simulink model "s_spg_pp"  (Simulink 8.1)
settings: Solver=ode4  SolverMode=SingleTasking  StartTime=0.0  StopTime=15  FixedStep=0.002  RelTol=1e-3  AbsTol=1e-6
values from neighbouring files (symbols this model uses):
  Beq = 5.4    [setup_ip01_2_configuration.m]
  Eff_g = 1    [setup_ip01_2_configuration.m]
  Eff_m = 1    [setup_ip01_2_configuration.m]
  IMAX_UPM = 3    [setup_ip01_2_configuration.m]
  K = place( A, B, cl_poles )    [d_ip02_spg_pp.m]    (also in prelab2_k_values.m = place (Ai,Bi,[p1, p2, p3, p4, p5]); setup_lab_ip02_spg.m = [ 0 0 0 0 ])
  Kg = 3.71    [setup_ip01_2_configuration.m]
  Km = 0.804e-3 * K_RDPS2RPM    [setup_ip01_2_configuration.m]
  Kt = 1.088 * K_OZ2N * K_IN2M    [setup_ip01_2_configuration.m]
  Mc = Mc + Eff_g * Kg^2 * Jm / r_mp^2    [setup_lab_ip02_spg.m]
  r_mp = 0.5 / 2 * K_IN2M    [setup_ip01_2_configuration.m]
  Rm = 2.6    [setup_ip01_2_configuration.m]
  VMAX_UPM = 13    [setup_ip01_2_configuration.m]
  X0 = [ 0; X0(2); 0; 0 ]    [setup_lab_ip02_spg.m]
undefined symbols (not defined in the file or in its folder): Bp, g, Ip, lp, Lp, Mp
libraries: simulink_extras x1
settings Model: Creator=Willdog  LastModifiedBy=Willdog  ExtModeArmWhenConnect=off  ExtModeAutoUpdateStatusClock=off  BufferReuse=off
settings DataIOCC: LimitDataPoints=off
settings OptimizationCC: BooleanDataType=off  OptimizeBlockIOStorage=off  BufferReuse=off  ExpressionFolding=off  ExpressionDepthLimit=128  FoldNonRolledExpr=off  LocalBlockOutputs=off  InitFltsAndDblsToZero=on
settings DebuggingCC: SaveWithParameterizedLinksMsg=none  SignalResolutionControl=TryResolveAllWithWarning  SolverPrmCheckMsg=none  MultiTaskDSMMsg=warning  MultiTaskCondExecSysMsg=none  StrictBusMsg=None
settings RTWCC: SystemTargetFile=wincon.tlc  MakeCommand=make_wc  TemplateMakefile=nt_msvc.tmf  Description=WinCon Target  ProcessScript=wincon_make_rtw_hook  IncludeERTFirstTime=on
settings STFCustomTargetCC: TargetFcnLib=ansi_tfl_tmw.mat  CodeReplacementLibrary=ANSI_C  ModelReferenceCompliant=off  GeneratePreprocessorConditionals=Disable all  SystemTargetFile=wincon.tlc
settings GRTTargetCC: TargetFcnLib=ansi_tfl_tmw.mat  ModelReferenceCompliant=off  ParMdlRefBuildCompliant=off  CompOptLevelCompliant=off  ConcurrentExecutionCompliant=off  MatFileLogging=off  ExtMode=on
settings CustomProperty: Value=on

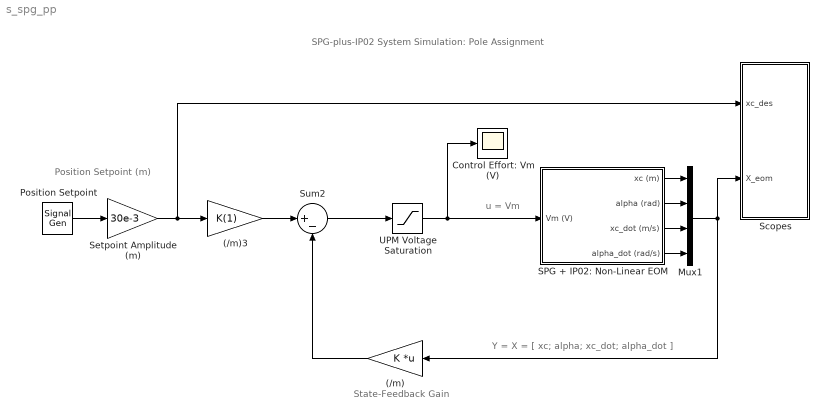
== system s_spg_pp ==
  note: u = Vm
  note: Y = X = [ xc; alpha; xc_dot; alpha_dot ]
  note: State-Feedback Gain
  note: Position Setpoint (m)
  note: SPG-plus-IP02 System Simulation:
      | Pole Assignment
  (/m) : Gain  Gain=K  Multiplication=Matrix(K*u)  SaturateOnIntegerOverflow=on  OutDataTypeStr=Inherit: Same as input  ParamDataTypeStr=Inherit: Same as input
  (/m)3 : Gain  Gain=K(1)  SaturateOnIntegerOverflow=on  OutDataTypeStr=Inherit: Same as input  ParamDataTypeStr=Inherit: Same as input
  Control Effort: Vm (V) : Scope
      settings: TickLabels=on  TimeRange=5  YMin=-35  YMax=35  SaveName=ScopeData2
  Mux1 : Mux
  Position Setpoint : SignalGenerator  WaveForm=square  Amplitude=0  Frequency=0.1
  SPG + IP02: Non-Linear EOM : Subsystem
  Scopes : Subsystem
  Setpoint Amplitude (m) : Gain  Gain=30e-3  SaturateOnIntegerOverflow=on  OutDataTypeStr=Inherit: Same as input  ParamDataTypeStr=Inherit: Same as input
  Sum2 : Sum  Inputs=|+-  SaturateOnIntegerOverflow=on  InputSameDT=on  OutDataTypeStr=Inherit: Same as first input
  UPM Voltage Saturation : Saturate  UpperLimit=VMAX_UPM  LowerLimit=- VMAX_UPM
  wires:
  UPM Voltage Saturation/1 -> Control Effort: Vm (V)/1, SPG + IP02: Non-Linear EOM/1(Vm (V))
  (/m)3/1 -> Sum2/1
  Setpoint Amplitude (m)/1 -> Scopes/1(xc_des), (/m)3/1
  Position Setpoint/1 -> Setpoint Amplitude (m)/1
  Mux1/1 -> Scopes/2(X_eom), (/m)/1
  (/m)/1 -> Sum2/2
  SPG + IP02: Non-Linear EOM/1(xc (m)) -> Mux1/1
  SPG + IP02: Non-Linear EOM/2(alpha (rad)) -> Mux1/2
  SPG + IP02: Non-Linear EOM/3(xc_dot (m/s)) -> Mux1/3
  SPG + IP02: Non-Linear EOM/4(alpha_dot (rad/s)) -> Mux1/4
  Sum2/1 -> UPM Voltage Saturation/1

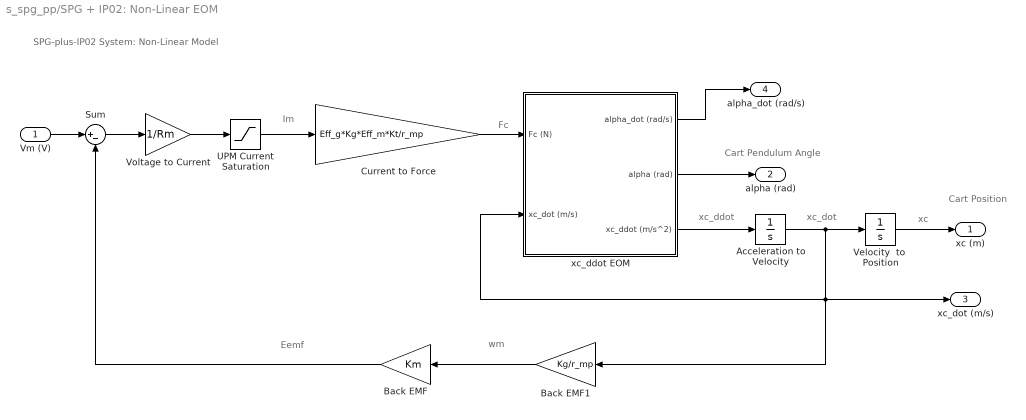
== system s_spg_pp/SPG + IP02: Non-Linear EOM ==
  note: SPG-plus-IP02 System:
      | Non-Linear Model
  note: Fc
  note: Im
  note: Eemf
  note: wm
  note: xc_dot
  note: xc_ddot
  note: xc
  note: Cart Position
  note: Cart Pendulum Angle
  Vm (V) : Inport
  Acceleration to Velocity : Integrator  InitialCondition=X0(3)
  Back EMF : Gain  Gain=Km  SaturateOnIntegerOverflow=on  OutDataTypeStr=Inherit: Same as input  ParamDataTypeStr=Inherit: Same as input
  Back EMF1 : Gain  Gain=Kg/r_mp  SaturateOnIntegerOverflow=on  OutDataTypeStr=Inherit: Same as input  ParamDataTypeStr=Inherit: Same as input
  Current to Force : Gain  Gain=Eff_g*Kg*Eff_m*Kt/r_mp  SaturateOnIntegerOverflow=on  OutDataTypeStr=Inherit: Same as input  ParamDataTypeStr=Inherit: Same as input
  Sum : Sum  Inputs=|+-  SaturateOnIntegerOverflow=on  InputSameDT=on  OutDataTypeStr=Inherit: Same as first input
  "UPM Current Saturation " : Saturate  UpperLimit=IMAX_UPM  LowerLimit=- IMAX_UPM
  Velocity  to  Position : Integrator  InitialCondition=X0(1)
  Voltage to Current : Gain  Gain=1/Rm  SaturateOnIntegerOverflow=on  OutDataTypeStr=Inherit: Same as input  ParamDataTypeStr=Inherit: Same as input
  xc_ddot EOM : Subsystem
  xc (m) : Outport
  alpha (rad) : Outport  Port=2
  xc_dot (m/s) : Outport  Port=3  InitialOutput=0
  alpha_dot (rad/s) : Outport  Port=4  InitialOutput=0
  wires:
  Sum/1 -> Voltage to Current/1
  Voltage to Current/1 -> "UPM Current Saturation "/1
  Acceleration to Velocity/1 -> xc_dot (m/s)/1, Back EMF1/1, xc_ddot EOM/2(xc_dot (m/s)), Velocity  to  Position/1
  Back EMF1/1 -> Back EMF/1
  Vm (V)/1 -> Sum/1
  Velocity  to  Position/1 -> xc (m)/1
  Back EMF/1 -> Sum/2
  "UPM Current Saturation "/1 -> Current to Force/1
  Current to Force/1 -> xc_ddot EOM/1(Fc (N))
  xc_ddot EOM/3(xc_ddot (m/s^2)) -> Acceleration to Velocity/1
  xc_ddot EOM/2(alpha (rad)) -> alpha (rad)/1
  xc_ddot EOM/1(alpha_dot (rad/s)) -> alpha_dot (rad/s)/1

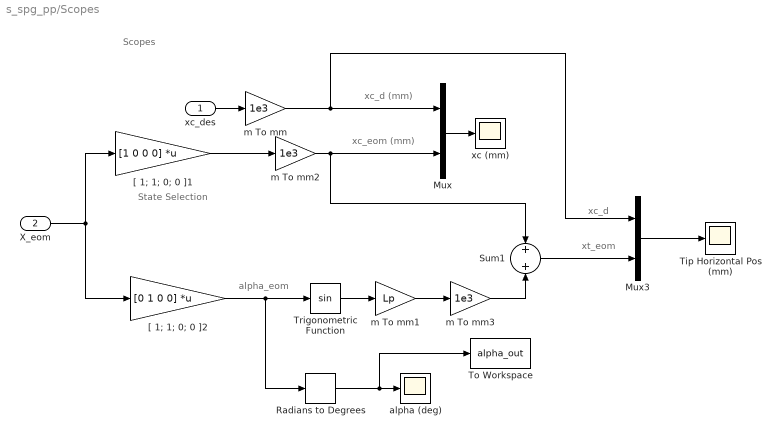
== system s_spg_pp/Scopes ==
  note: Scopes
  note: xc_d (mm)
  note: alpha_eom
  note: State Selection
  note: xc_eom (mm)
  note: xc_d
  note: xt_eom
  xc_des : Inport
  X_eom : Inport  Port=2
  Mux : Mux  Inputs=2
  Mux3 : Mux  Inputs=2
  Radians to Degrees : simulink_extras/Transformations/Radians to Degrees
  Sum1 : Sum  Inputs=+|+  SaturateOnIntegerOverflow=on  InputSameDT=on  OutDataTypeStr=Inherit: Same as first input
  Tip Horizontal Pos (mm) : Scope
      settings: SaveName=ScopeData5
  To Workspace : ToWorkspace  VariableName=alpha_out  SampleTime=-1  SaveFormat=Timeseries
  Trigonometric Function : Trigonometry
  "[ 1; 1; 0; 0 ]1" : Gain  Gain=[1 0 0 0]  Multiplication=Matrix(K*u)  SaturateOnIntegerOverflow=on  OutDataTypeStr=Inherit: Same as input  ParamDataTypeStr=Inherit: Same as input
  "[ 1; 1; 0; 0 ]2" : Gain  Gain=[0 1 0 0]  Multiplication=Matrix(K*u)  SaturateOnIntegerOverflow=on  OutDataTypeStr=Inherit: Same as input  ParamDataTypeStr=Inherit: Same as input
  alpha (deg) : Scope
      settings: TickLabels=on  TimeRange=1.000000  YMin=-250  YMax=250  SaveName=ScopeData3
  m To mm : Gain  Gain=1e3  SaturateOnIntegerOverflow=on  OutDataTypeStr=Inherit: Same as input  ParamDataTypeStr=Inherit: Same as input
  m To mm1 : Gain  Gain=Lp  SaturateOnIntegerOverflow=on  OutDataTypeStr=Inherit: Same as input  ParamDataTypeStr=Inherit: Same as input
  m To mm2 : Gain  Gain=1e3  SaturateOnIntegerOverflow=on  OutDataTypeStr=Inherit: Same as input  ParamDataTypeStr=Inherit: Same as input
  m To mm3 : Gain  Gain=1e3  SaturateOnIntegerOverflow=on  OutDataTypeStr=Inherit: Same as input  ParamDataTypeStr=Inherit: Same as input
  xc (mm) : Scope
      settings: TickLabels=on  TimeRange=5  YMin=-35  YMax=35
  wires:
  "[ 1; 1; 0; 0 ]2"/1 -> Radians to Degrees/1, Trigonometric Function/1
  X_eom/1 -> "[ 1; 1; 0; 0 ]2"/1, "[ 1; 1; 0; 0 ]1"/1
  xc_des/1 -> m To mm/1
  "[ 1; 1; 0; 0 ]1"/1 -> m To mm2/1
  Mux/1 -> xc (mm)/1
  m To mm1/1 -> m To mm3/1
  Trigonometric Function/1 -> m To mm1/1
  m To mm3/1 -> Sum1/2
  Radians to Degrees/1 -> To Workspace/1, alpha (deg)/1
  Mux3/1 -> Tip Horizontal Pos (mm)/1
  Sum1/1 -> Mux3/2
  m To mm/1 -> Mux/1, Mux3/1
  m To mm2/1 -> Mux/2, Sum1/1

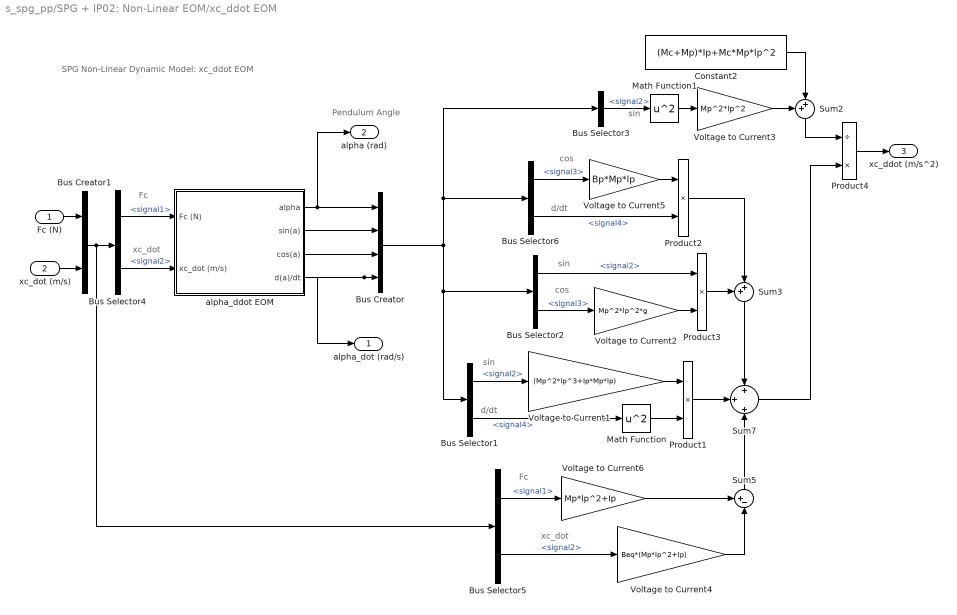
== system s_spg_pp/SPG + IP02: Non-Linear EOM/xc_ddot EOM ==
  note: d/dt
  note: sin
  note: sin
  note: cos
  note: sin
  note: Pendulum Angle
  note: cos
  note: d/dt
  note: Fc
  note: xc_dot
  note: Fc
  note: xc_dot
  note: SPG Non-Linear Dynamic Model:
      | xc_ddot EOM
  Fc (N) : Inport
  xc_dot (m/s) : Inport  Port=2
  Bus Creator : BusCreator
  Bus Creator1 : BusCreator  Inputs=2
  Bus Selector1 : BusSelector  OutputSignals=signal2,signal4
  Bus Selector2 : BusSelector  OutputSignals=signal2,signal3
  Bus Selector3 : BusSelector  OutputSignals=signal2
  Bus Selector4 : BusSelector  OutputSignals=signal1,signal2
  Bus Selector5 : BusSelector  OutputSignals=signal1,signal2
  Bus Selector6 : BusSelector  OutputSignals=signal3,signal4
  Constant2 : Constant  Value=(Mc+Mp)*Ip+Mc*Mp*lp^2
  Math Function : Math  Operator=square  SaturateOnIntegerOverflow=on
  Math Function1 : Math  Operator=square  SaturateOnIntegerOverflow=on
  Product1 : Product  SaturateOnIntegerOverflow=on  RndMeth=Zero  InputSameDT=on  OutDataTypeStr=Inherit: Same as first input
  Product2 : Product  SaturateOnIntegerOverflow=on  RndMeth=Zero  InputSameDT=on  OutDataTypeStr=Inherit: Same as first input
  Product3 : Product  SaturateOnIntegerOverflow=on  RndMeth=Zero  InputSameDT=on  OutDataTypeStr=Inherit: Same as first input
  Product4 : Product  Inputs=/*  SaturateOnIntegerOverflow=on  RndMeth=Zero  InputSameDT=on  OutDataTypeStr=Inherit: Same as first input
  Sum2 : Sum  Inputs=++|  SaturateOnIntegerOverflow=on  InputSameDT=on  OutDataTypeStr=Inherit: Same as first input
  Sum3 : Sum  Inputs=++|  SaturateOnIntegerOverflow=on  InputSameDT=on  OutDataTypeStr=Inherit: Same as first input
  Sum5 : Sum  Inputs=+-|  SaturateOnIntegerOverflow=on  InputSameDT=on  OutDataTypeStr=Inherit: Same as first input
  Sum7 : Sum  Inputs=+|+|+  SaturateOnIntegerOverflow=on  InputSameDT=on  OutDataTypeStr=Inherit: Same as first input
  Voltage to Current1 : Gain  Gain=(Mp^2*lp^3+Ip*Mp*lp)  SaturateOnIntegerOverflow=on  OutDataTypeStr=Inherit: Same as input  ParamDataTypeStr=Inherit: Same as input
  Voltage to Current2 : Gain  Gain=Mp^2*lp^2*g  SaturateOnIntegerOverflow=on  OutDataTypeStr=Inherit: Same as input  ParamDataTypeStr=Inherit: Same as input
  Voltage to Current3 : Gain  Gain=Mp^2*lp^2  SaturateOnIntegerOverflow=on  OutDataTypeStr=Inherit: Same as input  ParamDataTypeStr=Inherit: Same as input
  Voltage to Current4 : Gain  Gain=Beq*(Mp*lp^2+Ip)  SaturateOnIntegerOverflow=on  OutDataTypeStr=Inherit: Same as input  ParamDataTypeStr=Inherit: Same as input
  Voltage to Current5 : Gain  Gain=Bp*Mp*lp  SaturateOnIntegerOverflow=on  OutDataTypeStr=Inherit: Same as input  ParamDataTypeStr=Inherit: Same as input
  Voltage to Current6 : Gain  Gain=Mp*lp^2+Ip  SaturateOnIntegerOverflow=on  OutDataTypeStr=Inherit: Same as input  ParamDataTypeStr=Inherit: Same as input
  alpha_ddot EOM : Subsystem
  alpha_dot (rad/s) : Outport
  alpha (rad) : Outport  Port=2
  xc_ddot (m/s^2) : Outport  Port=3
  wires:
  Sum2/1 -> Product4/1
  Bus Creator/1 -> Bus Selector2/1, Bus Selector1/1, Bus Selector3/1, Bus Selector6/1
  Voltage to Current1/1 -> Product1/1
  Math Function/1 -> Product1/2
  Voltage to Current2/1 -> Product3/2
  Bus Selector3/1 -> Math Function1/1  "<signal2>"
  Math Function1/1 -> Voltage to Current3/1
  Voltage to Current3/1 -> Sum2/1
  Constant2/1 -> Sum2/2
  Product1/1 -> Sum7/2
  Product4/1 -> xc_ddot (m/s^2)/1
  alpha_ddot EOM/1(alpha) -> Bus Creator/1, alpha (rad)/1
  alpha_ddot EOM/2(sin(a)) -> Bus Creator/2
  alpha_ddot EOM/3(cos(a)) -> Bus Creator/3
  alpha_ddot EOM/4(d(a)/dt) -> Bus Creator/4, alpha_dot (rad/s)/1
  Fc (N)/1 -> Bus Creator1/1
  xc_dot (m/s)/1 -> Bus Creator1/2
  Bus Creator1/1 -> Bus Selector4/1, Bus Selector5/1
  Bus Selector4/1 -> alpha_ddot EOM/1(Fc (N))  "<signal1>"
  Bus Selector4/2 -> alpha_ddot EOM/2(xc_dot (m/s))  "<signal2>"
  Bus Selector1/2 -> Math Function/1  "<signal4>"
  Bus Selector1/1 -> Voltage to Current1/1  "<signal2>"
  Bus Selector6/1 -> Voltage to Current5/1  "<signal3>"
  Bus Selector6/2 -> Product2/2  "<signal4>"
  Bus Selector2/1 -> Product3/1  "<signal2>"
  Bus Selector2/2 -> Voltage to Current2/1  "<signal3>"
  Voltage to Current5/1 -> Product2/1
  Bus Selector5/1 -> Voltage to Current6/1  "<signal1>"
  Bus Selector5/2 -> Voltage to Current4/1  "<signal2>"
  Sum7/1 -> Product4/2
  Product2/1 -> Sum3/2
  Product3/1 -> Sum3/1
  Sum3/1 -> Sum7/1
  Sum5/1 -> Sum7/3
  Voltage to Current6/1 -> Sum5/1
  Voltage to Current4/1 -> Sum5/2

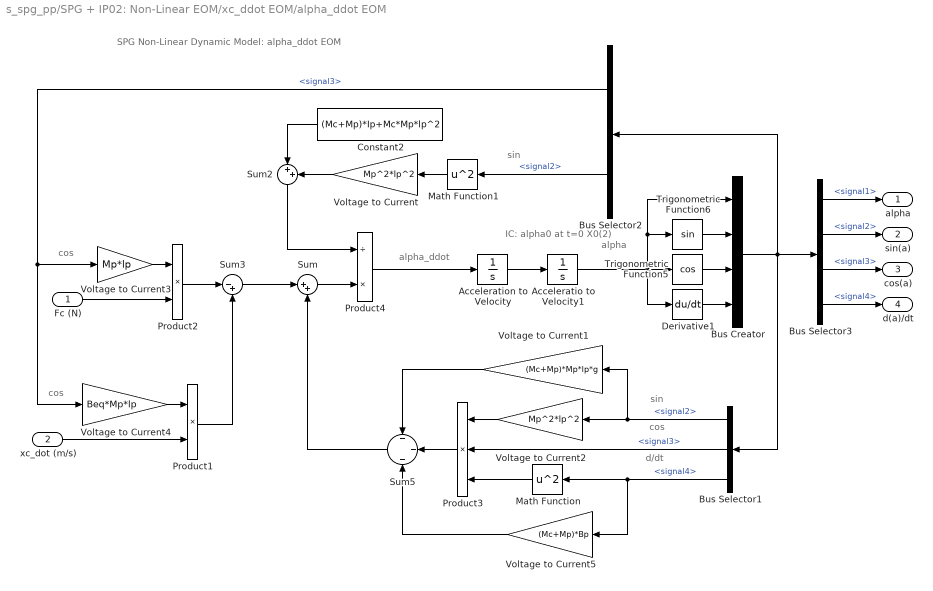
== system s_spg_pp/SPG + IP02: Non-Linear EOM/xc_ddot EOM/alpha_ddot EOM ==
  note: d/dt
  note: cos
  note: sin
  note: cos
  note: sin
  note: alpha
  note: IC: alpha0 at t=0
      | X0(2)
  note: alpha_ddot
  note: cos
  note: SPG Non-Linear Dynamic Model:
      | alpha_ddot EOM
  Fc (N) : Inport
  xc_dot (m/s) : Inport  Port=2
  Acceleratio to Velocity1 : Integrator  InitialCondition=X0(2)
  Acceleration to Velocity : Integrator  InitialCondition=X0(4)
  Bus Creator : BusCreator
  Bus Selector1 : BusSelector  OutputSignals=signal2,signal3,signal4
  Bus Selector2 : BusSelector  OutputSignals=signal3,signal2
  Bus Selector3 : BusSelector  OutputSignals=signal1,signal2,signal3,signal4
  Constant2 : Constant  Value=(Mc+Mp)*Ip+Mc*Mp*lp^2
  Derivative1 : Derivative
  Math Function : Math  Operator=square  SaturateOnIntegerOverflow=on
  Math Function1 : Math  Operator=square  SaturateOnIntegerOverflow=on
  Product1 : Product  SaturateOnIntegerOverflow=on  RndMeth=Zero  InputSameDT=on  OutDataTypeStr=Inherit: Same as first input
  Product2 : Product  SaturateOnIntegerOverflow=on  RndMeth=Zero  InputSameDT=on  OutDataTypeStr=Inherit: Same as first input
  Product3 : Product  Inputs=3  SaturateOnIntegerOverflow=on  RndMeth=Zero  InputSameDT=on  OutDataTypeStr=Inherit: Same as first input
  Product4 : Product  Inputs=/*  SaturateOnIntegerOverflow=on  RndMeth=Zero  InputSameDT=on  OutDataTypeStr=Inherit: Same as first input
  Sum : Sum  Inputs=|++  SaturateOnIntegerOverflow=on  InputSameDT=on  OutDataTypeStr=Inherit: Same as first input
  Sum2 : Sum  Inputs=|++  SaturateOnIntegerOverflow=on  InputSameDT=on  OutDataTypeStr=Inherit: Same as first input
  Sum3 : Sum  Inputs=|-+  SaturateOnIntegerOverflow=on  InputSameDT=on  OutDataTypeStr=Inherit: Same as first input
  Sum5 : Sum  Inputs=-|-|-  SaturateOnIntegerOverflow=on  InputSameDT=on  OutDataTypeStr=Inherit: Same as first input
  Trigonometric Function5 : Trigonometry  Operator=cos
  Trigonometric Function6 : Trigonometry
  Voltage to Current : Gain  Gain=Mp^2*lp^2  SaturateOnIntegerOverflow=on  OutDataTypeStr=Inherit: Same as input  ParamDataTypeStr=Inherit: Same as input
  Voltage to Current1 : Gain  Gain=(Mc+Mp)*Mp*lp*g  SaturateOnIntegerOverflow=on  OutDataTypeStr=Inherit: Same as input  ParamDataTypeStr=Inherit: Same as input
  Voltage to Current2 : Gain  Gain=Mp^2*lp^2  SaturateOnIntegerOverflow=on  OutDataTypeStr=Inherit: Same as input  ParamDataTypeStr=Inherit: Same as input
  Voltage to Current3 : Gain  Gain=Mp*lp  SaturateOnIntegerOverflow=on  OutDataTypeStr=Inherit: Same as input  ParamDataTypeStr=Inherit: Same as input
  Voltage to Current4 : Gain  Gain=Beq*Mp*lp  SaturateOnIntegerOverflow=on  OutDataTypeStr=Inherit: Same as input  ParamDataTypeStr=Inherit: Same as input
  Voltage to Current5 : Gain  Gain=(Mc+Mp)*Bp  SaturateOnIntegerOverflow=on  OutDataTypeStr=Inherit: Same as input  ParamDataTypeStr=Inherit: Same as input
  alpha : Outport  InitialOutput=0
  sin(a) : Outport  Port=2  InitialOutput=0
  cos(a) : Outport  Port=3  InitialOutput=0
  d(a)/dt : Outport  Port=4  InitialOutput=0
  wires:
  Acceleration to Velocity/1 -> Acceleratio to Velocity1/1
  Bus Selector1/1 -> Voltage to Current1/1, Voltage to Current2/1  "<signal2>"
  Product4/1 -> Acceleration to Velocity/1
  Math Function/1 -> Product3/3
  Sum2/1 -> Product4/1
  Sum/1 -> Product4/2
  Voltage to Current/1 -> Sum2/2
  Bus Selector2/2 -> Math Function1/1  "<signal2>"
  Math Function1/1 -> Voltage to Current/1
  Constant2/1 -> Sum2/1
  Trigonometric Function6/1 -> Bus Creator/2
  Trigonometric Function5/1 -> Bus Creator/3
  Derivative1/1 -> Bus Creator/4
  Bus Creator/1 -> Bus Selector2/1, Bus Selector1/1, Bus Selector3/1
  Bus Selector2/1 -> Voltage to Current3/1, Voltage to Current4/1  "<signal3>"
  Voltage to Current2/1 -> Product3/1
  Bus Selector1/2 -> Product3/2  "<signal3>"
  Bus Selector1/3 -> Math Function/1, Voltage to Current5/1  "<signal4>"
  Bus Selector3/1 -> alpha/1  "<signal1>"
  Bus Selector3/2 -> sin(a)/1  "<signal2>"
  Bus Selector3/3 -> cos(a)/1  "<signal3>"
  Bus Selector3/4 -> d(a)/dt/1  "<signal4>"
  Acceleratio to Velocity1/1 -> Trigonometric Function5/1, Derivative1/1, Trigonometric Function6/1, Bus Creator/1
  Voltage to Current3/1 -> Product2/1
  Fc (N)/1 -> Product2/2
  xc_dot (m/s)/1 -> Product1/2
  Voltage to Current4/1 -> Product1/1
  Product2/1 -> Sum3/1
  Product1/1 -> Sum3/2
  Sum3/1 -> Sum/1
  Product3/1 -> Sum5/2
  Voltage to Current1/1 -> Sum5/1
  Voltage to Current5/1 -> Sum5/3
  Sum5/1 -> Sum/2
